simulink model "Level1"  (R2021a)
settings: Solver=VariableStepAuto  StartTime=0.0  StopTime=10.0  RelTol=1e-3
values from neighbouring files (symbols this model uses):
  ax_max = 0.8    [Data.m]
  ay_max = 0.75    [Data.m]
  Bseg = 2    [Data.m]
  containerLayout = [3 2 2 4 3 4 2 1 4]    [Data.m]
  containerWidth = 2.5    [Data.m]
  dx = 0.1    [Data.m]    (also in generate_profile.m)
  Hseg = 3    [Data.m]
  jerkh = 4    [Data.m]
  jerkt = 2    [Data.m]
  vx_max = 4    [Data.m]
  vy_loaded_max = 1.5    [Data.m]
  vy_unloaded_max = 3    [Data.m]
  x_axis = [-30 50]    [Data.m]
  X_bay = [-22,-15,-8]    [Data.m]
  X_container = [2.8,5.4,8,10.6,13.2,15.8,18.4,21,23.6]    [Data.m]
  y_axis = [-20 40]    [Data.m]
  Yt0 = 45    [Data.m]
libraries: simulink x1
settings Model: Creator=jpss8  LastModifiedBy=ThnkPad

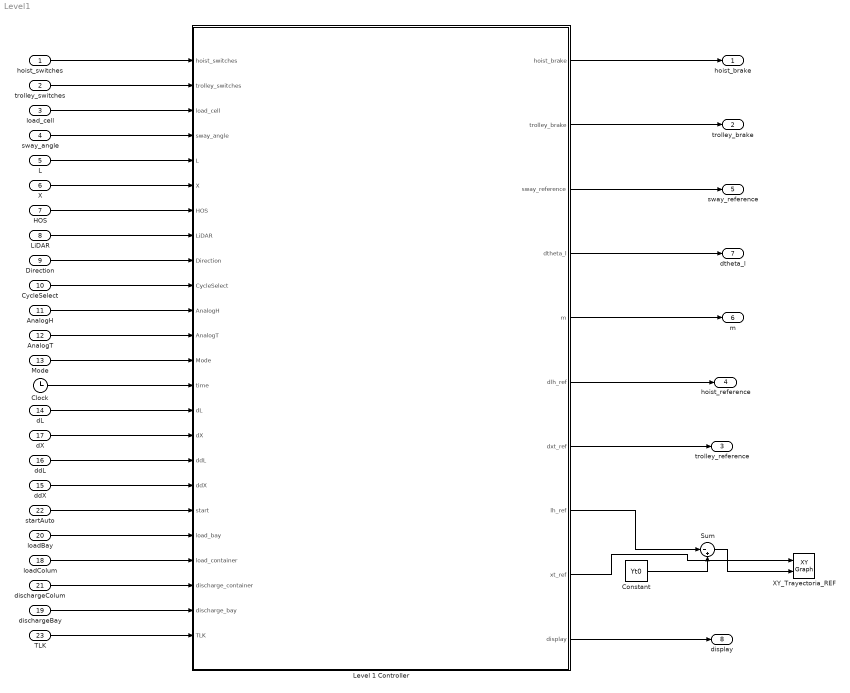
== system Level1 ==
  hoist_switches : Inport  PortDimensions=4
  trolley_switches : Inport  Port=2  PortDimensions=4
  load_cell : Inport  Port=3
  sway_angle : Inport  Port=4
  L : Inport  Port=5
  X : Inport  Port=6
  HOS : Inport  Port=7
  LiDAR : Inport  Port=8
  Direction : Inport  Port=9
  CycleSelect : Inport  Port=10
  AnalogH : Inport  Port=11
  AnalogT : Inport  Port=12
  Mode : Inport  Port=13
  dL : Inport  Port=14
  ddX : Inport  Port=15
  ddL : Inport  Port=16
  dX : Inport  Port=17
  loadColum : Inport  Port=18
  dischargeBay : Inport  Port=19
  loadBay : Inport  Port=20
  dischargeColum : Inport  Port=21
  startAuto : Inport  Port=22
  TLK : Inport  Port=23
  Clock : Clock
  Constant : Constant  Value=Yt0
  Level 1 Controller : Stateflow chart  TreatAsAtomicUnit=on
  Sum : Sum  Inputs=|-+
  XY_Trayectoria_REF : simulink/Sinks/XY Graph  xmin=-30  xmax=50  ymin=-20  ymax=45  st=-1
  hoist_brake : Outport
  trolley_brake : Outport  Port=2
  trolley_reference : Outport  Port=3
  hoist_reference : Outport  Port=4
  sway_reference : Outport  Port=5
  m : Outport  Port=6
  dtheta_l : Outport  Port=7
  display : Outport  Port=8
  wires:
  load_cell/1 -> Level 1 Controller/3(load_cell)
  sway_angle/1 -> Level 1 Controller/4(sway_angle)
  L/1 -> Level 1 Controller/5(L)
  Level 1 Controller/6(dlh_ref) -> hoist_reference/1
  Level 1 Controller/2(trolley_brake) -> trolley_brake/1
  Level 1 Controller/1(hoist_brake) -> hoist_brake/1
  Level 1 Controller/3(sway_reference) -> sway_reference/1
  HOS/1 -> Level 1 Controller/7(HOS)
  trolley_switches/1 -> Level 1 Controller/2(trolley_switches)
  hoist_switches/1 -> Level 1 Controller/1(hoist_switches)
  LiDAR/1 -> Level 1 Controller/8(LiDAR)
  Direction/1 -> Level 1 Controller/9(Direction)
  CycleSelect/1 -> Level 1 Controller/10(CycleSelect)
  AnalogH/1 -> Level 1 Controller/11(AnalogH)
  AnalogT/1 -> Level 1 Controller/12(AnalogT)
  Mode/1 -> Level 1 Controller/13(Mode)
  Level 1 Controller/5(m) -> m/1
  Level 1 Controller/4(dtheta_l) -> dtheta_l/1
  X/1 -> Level 1 Controller/6(X)
  Clock/1 -> Level 1 Controller/14(time)
  dL/1 -> Level 1 Controller/15(dL)
  Level 1 Controller/9(xt_ref) -> XY_Trayectoria_REF/1
  Sum/1 -> XY_Trayectoria_REF/2
  Level 1 Controller/8(lh_ref) -> Sum/1
  Constant/1 -> Sum/2
  Level 1 Controller/7(dxt_ref) -> trolley_reference/1
  dX/1 -> Level 1 Controller/16(dX)
  ddL/1 -> Level 1 Controller/17(ddL)
  ddX/1 -> Level 1 Controller/18(ddX)
  loadBay/1 -> Level 1 Controller/20(load_bay)
  loadColum/1 -> Level 1 Controller/21(load_container)
  dischargeColum/1 -> Level 1 Controller/22(discharge_container)
  dischargeBay/1 -> Level 1 Controller/23(discharge_bay)
  startAuto/1 -> Level 1 Controller/19(start)
  Level 1 Controller/10(display) -> display/1
  TLK/1 -> Level 1 Controller/24(TLK)

== stateflow chart Level1/Level 1 Controller ==
  state AutoSecuence [parallel]
    settings: executionOrder=3
    state stay
      entry:
      display=4;
      AUTO=0;
    state automaticSecuence
      state Positioning [group]
        state m1
          %manual hasta salir de manualZone
          entry:
          AUTO=0;
          display=0;
        state Pos
          entry:
          %ir hasta la bahia de carga seleccionada
          Xf=X_bay(discharge_bay);
          Yf=interp1(manualZone(1,:),manualZone(2,:), Xf, 'linear');
          AutoFlag=0;
          AUTO=1;
          display=1;
        state m2a
          entry:
          %tomar el container
          AUTO=0;
          display=2;
        m1 -> Pos : [MZF==0]
        Pos -> m2a : [AutoFlag==1]
      state go [group]
        state m2b
          %salir de la zona manual
          display=0;
        state Go
          entry:
          %ir hasta la culumna a cargar
          Xf=X_container(load_container);
          Yf=interp1(manualZone(1,:),manualZone(2,:), Xf, 'linear');
          AutoFlag=0;
          AUTO=1;
          display=1;
        state m3a
          entry:
          %soltar manualmente el container
          AUTO=0;
          display=3;
        m2b -> Go : [MZF==0]
        Go -> m3a : [AutoFlag==1]
      state Transit [group]
        state m3b
          %salir de la zona manual
          display=0;
        state Transist
          %ir hasta la columna de container a descargar
          entry:
          Xf=X_container(discharge_container);
          Yf=interp1(manualZone(1,:),manualZone(2,:), Xf, 'linear');
          AutoFlag=0;
          AUTO=1;
          display=1;
        state m4a
          %tomar el container manualmente
          entry:
          AUTO=0;
          display=2;
        AutoSecuence.automaticSecuence.Transit.m3b -> Transist : [MZF==0]
        Transist -> AutoSecuence.automaticSecuence.Transit.m4a : [AutoFlag==1]
      state Return [group]
        state m3b
          %salir de la zona manual para volver
          display=0;
        state Return
          %if hasta la bahia de carga a cargar
          entry:
          Xf=X_bay(load_bay);
          Yf=interp1(manualZone(1,:),manualZone(2,:), Xf, 'linear');
          AutoFlag=0;
          AUTO=1;
          display=1;
        state m4a
          entry:
          AUTO=0;
          display=3;
        AutoSecuence.automaticSecuence.Return.m3b -> AutoSecuence.automaticSecuence.Return.Return : [MZF==0]
        AutoSecuence.automaticSecuence.Return.Return -> AutoSecuence.automaticSecuence.Return.m4a : [AutoFlag==1]
      (default) -> m1
      m2a -> m2b : [TLK==1]
      m3a -> AutoSecuence.automaticSecuence.Transit.m3b : [TLK==0]
      AutoSecuence.automaticSecuence.Transit.m4a -> AutoSecuence.automaticSecuence.Return.m3b : [TLK==1]
    (default) -> stay
    automaticSecuence -> stay : [Mode==0]
    stay -> automaticSecuence : [Mode==1 && start==1]
  state ObstacleProfile [parallel]
    entry:
    obst_profile=ones(2,(x_axis(2)-x_axis(1))/dx+1);
    obst_profile(1,:)=[x_axis(1):dx:x_axis(2)];
    manualZone=obst_profile;
    obst_profile(2,:)=obst_profile(2,:)*15;%y_axis(2)-5;
    obst_profile=obsProfGen(containerLayout);%prueba!!!!!!!!!!!!!!!!!!!!!!!!!!!!!!!!!!!!!!!!!!!!!!!!!!!!!!
    MZF=1;
    k=1;
    during:
    if TLK==0
    while obst_profile(1,k+1)<X
    k=k+1;
    end
    while obst_profile(1,k-1)>X
    k=k-1;
    end
    obst_profile(2,k)=Yt0-LiDAR;
    end
    manualZone=ObsToManaualZone(Hseg,Bseg,obst_profile);
    if MZF==1
    if interp1(manualZone(1,:),manualZone(2,:), X, 'linear')+0.2<Yt0-L
    MZF=0;
    end
    else
    if interp1(manualZone(1,:),manualZone(2,:), X, 'linear')-0.2>Yt0-L
    MZF=1;
    end
    end
    settings: executionOrder=2
  state Main [parallel]
    settings: executionOrder=1
    state On
      entry:
      sway_reference = 0;
      m = 0;
      dtheta_l = 0;
      dxt_ref=0;
      dlh_ref=0;
    state Manual
      entry:
      AnalogH_1=0;
      jH=1;
      AnalogT_1=0;
      jT=1;
      t0H=time;
      t0T=time;
      if TLK==0
      vH_max=vy_unloaded_max;
      else
      vH_max=vy_loaded_max;
      end
      [t_H,v_H]= vel_prof_gen(-dL, -AnalogH*vH_max/100 , -ddL ,vH_max,ay_max, jerkh,0.0005);
      [t_T,v_T]= vel_prof_gen(dX, AnalogT*vx_max/100 , ddX ,vx_max,ax_max, jerkt,0.0005);
      during:
      %-----------------------HOIST---------------------------------------------------
      if abs(AnalogH-AnalogH_1)>abs(AnalogH)*0.01
      AnalogH_1=AnalogH;
      jH=1;
      t0H=time;
      if TLK==0
      vH_max=vy_unloaded_max;
      else
      vH_max=vy_loaded_max;
      end
      [t_H,v_H]= vel_prof_gen(-dL, -AnalogH*vH_max/100 , -ddL ,vH_max,ay_max, jerkh,0.0005);
      end
      if time>t0H+t_H(end)
      dlh_ref=-v_H(end);
      else
      while time>t_H(jH)+t0H
      jH=jH+1;
      end
      dlh_ref=-v_H(jH);
      end
      %------------------------TROLLEY---------------------------------------------
      if abs(AnalogT-AnalogT_1)>abs(AnalogT)*0.01
      AnalogT_1=AnalogT;
      jT=1;
      t0T=time;
      [t_T,v_T]= vel_prof_gen(dX, AnalogT*vx_max/100 , ddX ,vx_max,ax_max, jerkt,0.0005);
      end
      if time>t0T+t_T(end)
      dxt_ref=v_T(end);
      else
      while time>t_T(jT)+t0T
      jT=jT+1;
      end
      dxt_ref=v_T(jT);
      end
    state Automatic
      entry:
      Xf=X_bay(load_bay);
      Yf=interp1(manualZone(1,:),manualZone(2,:), Xf, 'linear');
      disp([X,Yt0-L])
      disp([Xf,Yf])
      disp(-dL)
      disp(vy_unloaded_max)
      disp(vx_max)
      disp(-ddL)
      if (TLK==0)
      [T_,Qhoist_,Qtrolley_]=traj_gen(obst_profile',[X,Yt0-L],[Xf,Yf],-dL,0,vy_unloaded_max,vx_max,0,0,ay_max,ax_max,jerkt,jerkh,containerWidth,Hseg);
      else
      [T_,Qhoist_,Qtrolley_]=traj_gen(obst_profile',[X,Yt0-L],[Xf,Yf],-dL,0,vy_loaded_max,vx_max,0,0,ay_max,ax_max,jerkt,jerkh,containerWidth,Hseg);
      end
      set(TrajP,'XData', Qtrolley_(1,:), 'YData', Qhoist_(1,:));
      t0=time;
      N=length(T_);
      i_=1;
      during:
      if time-t0>T_(end)
      AutoFlag=1;
      else
      while T_(i_)<time-t0
      i_=i_+1;
      end
      dlh_ref=-Qhoist_(2,i_);
      dxt_ref=Qtrolley_(2,i_);
      lh_ref=Yt0-Qhoist_(1,i_);
      xt_ref=Qtrolley_(1,i_);
      end
    (default) -> On
    On -> Manual
    Automatic -> Manual : [AUTO==0]
    Manual -> Automatic : [AUTO==1]
  state Breaks [parallel]
    during:
    if dxt_ref==0
    trolley_brake = 0;
    else
    trolley_brake = 0;
    end
    if dlh_ref==0
    hoist_brake = 0;
    else
    hoist_brake = 0;
    end
    settings: executionOrder=5
  note: ?
  state Plot [parallel]
    entry:
    close all;
    figure(1);
    h = plot(nan, nan);
    hold on;
    TrajP = plot(nan, nan,'r');
    p = plot(nan, nan, 'ro', 'MarkerFaceColor', 'r');
    ps = plot(nan, nan, 'ro', 'MarkerFaceColor', 'b');
    xlabel('Eje X');
    ylabel('Eje Y');
    title('Grafico XY Animado');
    xlim([-30, 50]);
    ylim([-20, 45]);
    during:
    set(h, 'XData', obst_profile(1,:), 'YData', obst_profile(2,:));
    set(p, 'XData', X, 'YData', Yt0);
    set(ps, 'XData', X, 'YData', Yt0-L);
    drawnow;
    settings: executionOrder=4
  data: ManualZone function_output; hseg function_input; bseg function_input; obsProfile function_input; O_profile function_input; P0 function_input; Pf function_input; v0h function_input; vfh function_input; vmaxh function_input; vmaxt function_input; a0h function_input; afh function_input; amaxh function_input; amaxt function_input; T function_output; Qhoist function_output; Qtrolley function_output; jt function_input; jh function_input; xbox function_input; hseg function_input; Ob_profile function_output; Layout function_input; v0 function_input; vc function_input; a0 function_input; v_max function_input; a_max function_input; J function_input; dt function_input; t function_output; v function_output; hoist_brake output; trolley_brake output; hoist_switches input; trolley_switches input; load_cell input; sway_angle input; L input; X input; sway_reference output; dtheta_l output; HOS input; LiDAR input; Direction input; CycleSelect input; AnalogH input; AnalogT input; Mode input; m output; time input; t0 local; vy_loaded_max parameter; vy_unloaded_max parameter; ax_max parameter; vx_max parameter; ay_max parameter; dL input; i local; obst_profile local size=[2 801]; Qtrolley_ local size=[4 10000000]; T_ local size=[1 10000000]; Qhoist_ local size=[4 10000000]; jerkh parameter; jerkt parameter; containerWidth parameter; Hseg parameter; Yt0 parameter; dlh_ref output; dxt_ref output; lh_ref output; xt_ref output; N local; dX input; al_1 local; ax_1 local; t_1 local; Dt local; ddL input; ddX input; a_H local; a_T local; jT local; jH local; t0H local; vH_max local; t_H local size=10000000; v_H local size=10000000; t0T local; t_T local size=10000000; v_T local size=10000000; AnalogH_1 local; AnalogT_1 local; start input; X_bay parameter; load_bay input; dx parameter; x_axis parameter; y_axis parameter; load_container input; discharge_container input; X_container parameter; discharge_bay input; display output int8; manualZone local size=[2 801]; Xf local; Yf local; AutoFlag local; MZF local; Bseg parameter; AUTO local; TLK input; k local; i_ local; h local; containerLayout parameter size=9; p local; TrajP local; ps local
  function ManualZone=ObsToManaualZone(hseg,bseg,obsProfile):
    | function ManualZone=ObsToManaualZone(hseg,bseg,obsProfile)
    | 
    | ManualZone=obsProfile;
    | ManualZone(2,:)=obsProfile(2,:)+hseg;
    | 
    | N=round(bseg/(obsProfile(1,2)-obsProfile(1,1)));
    | 
    | for i=1:N
    |     ManualZone(2,i)=max(obsProfile(2,1:i+N)); 
    | end
    | for i=1+N:length(obsProfile(2,:))-N
    |     ManualZone(2,i)=max(obsProfile(2,i-N:i+N)); 
    | end
    | for i=length(obsProfile(2,:))-N+1:length(obsProfile(2,:))
    |     ManualZone(2,i)=max(obsProfile(2,i-N:end)); 
    | end
    | 
    | ManualZone(2,:)=ManualZone(2,:)+hseg;
    | 
    | end
  function [T,Qhoist,Qtrolley]=traj_gen(O_profile,P0,Pf,v0h,vfh,vmaxh,vmaxt,a0h,afh,amaxh,amaxt,jt,jh,xbox,hseg):
    | 
    | 
    | function [T,Qhoist,Qtrolley]=traj_gen(O_profile,P0,Pf,v0h,vfh,vmaxh,vmaxt,a0h,afh,amaxh,amaxt,jt,jh,xbox,hseg)
    | % Esta función genera una trayectoria para un sistema de elevación, como un
    | % montacargas o una grúa, en función de un perfil de elevación dado. 
    | % La trayectoria contempla aceleración con perfil trapeziodal.
    | % Busca generar una trayectoria eficiente donde evite los obstaculos con un
    | % marquen dado.
    | % Además admite casos donde la la aceleracion maxima o la velocidad maxima sean
    | % mayores a las posible para un determinado recorrido. Estos casos de
    | % diminuye automaticamente su valor para cumplir con los otros
    | % requirimientos.
    | %
    | % Argumentos de entrada:
    | % - O_profile: matriz que contiene el perfil de elevación. Cada fila representa
    | %   un punto en el perfil, donde la primera columna contiene las coordenadas
    | %   horizontales y la segunda columna contiene las alturas correspondientes.
    | % - P0: punto inicial de la trayectoria, dado como [x0, y0].
    | % - Pf: punto final de la trayectoria, dado como [xf, yf].
    | % - v0h: velocidad inicial de elevación.
    | % - vfh: velocidad final de elevación.
    | % - vmaxh: velocidad máxima de elevación.
    | % - vmaxt: velocidad máxima de desplazamiento horizontal.
    | % - a0h: aceleración inicial de elevación.
    | % - afh: aceleración final de elevación.
    | % - amaxh: aceleración máxima de elevación.
    | % - amaxt: aceleración máxima de desplazamiento horizontal.
    | %
    | % Las siguientes variables se toman del espacio de trabajo (workspace):
    | % - hseg: altura de seguridad adicional a considerar.
    | % - xbox: distancia horizontal alrededor de los puntos iniciales y finales
    | %   para buscar el perfil.
    | % - jh: jerk máximo permitido en la elevación.
    | % - jt: jerk máximo permitido en el desplazamiento horizontal.
    | %
    | % Argumentos de salida:
    | % - T: vector de tiempo de la trayectoria generada.
    | % - Qhoist: matriz que describe la trayectoria de elevación generada.
    | %   Siento las filas Q(1,:) la posición, Q(2,:) la velocidad,
    | %   Q(3,:)aceleracion y Q(4,:) el jerk
    | % - Qtrolley: matriz que describe la trayectoria de desplazamiento horizontal
    | %   generada. misma estructura que Qtrolley
    |     
    |     
    |     %Caso degenerado=======================================================
    |     if P0(1)==Pf(1)
    |         [T,Qhoist] = trap_acc_prof(P0(2),Pf(2),v0h,0,a0h,0,vmaxh,amaxh,jh);
    |         Qtrolley=zeros(4,length(T));
    |         Qtrolley(1,:)=ones(1,length(T))*P0(1);
    |         return;
    |     end  
    | 
    |     %=========================================================================
    |     %Calculo de puntos
    |     %=========================================================================
    |     %recortar O_profile entre x0 y xf (O_profile_r)
    |     O_profile_r=subO_profile(O_profile,P0(1),Pf(1));
    | 
    |     %Hmax es igual a la altula maxima en O_profile_r mas una altura de seguridad "h_seg"
    |     Hmax=max(O_profile_r(:,2))+hseg;
    | 
    |     %H0 es la altura que parte de Y0 y termina cuando el O_profile es superado en
    |     %un entorno de 1.5 xbox de X0 mas h_seg.
    |     H0=max(subO_profile(O_profile,P0(1)-xbox*1.5,P0(1)+xbox*1.5))+hseg;
    |     H0=H0(2);
    |     %H1 lo mismo
    |     Hf=max(subO_profile(O_profile,Pf(1)-xbox*1.5,Pf(1)+xbox*1.5))+hseg;
    |     Hf=Hf(2);
    |     %se traza una recta entre xo y el se la hace "tangente" (que solo toca un 
    |     %punto del O_profile)
    | 
    |     if Pf(1)>P0(1)
    |         xl=P0(1);
    |         xh=Pf(1);
    |         Hl=H0;
    |         Hh=Hf;
    |     else
    |         xh=P0(1);
    |         xl=Pf(1);
    |         Hh=H0;
    |         Hl=Hf;
    |     end
    | 
    |     mmax=0;
    |     prof=subO_profile(O_profile,xl+xbox*0.5,inf);
    |     for i=1:length(prof)
    |         if prof(i,2)+hseg<Hl
    |             continue
    |         end
    |         if (prof(i,2)+hseg-Hl)/(prof(i,1)-xbox-xl(1))>mmax
    |             mmax=(prof(i,2)-Hl+hseg)/(prof(i,1)-xl(1)-xbox);
    |         end
    |     end
    |     DXl=(Hmax-Hl)/mmax;
    | 
    |     mmax=0;
    |     prof=subO_profile(O_profile,xh-xbox*0.5,-inf);
    |     for i=1:length(prof)
    |         if prof(i,2)+hseg<Hh
    |             continue
    |         end
    |         if (prof(i,2)+hseg-Hh)/(prof(i,1)+xbox-xh(1))<mmax
    |             mmax=(prof(i,2)-Hh+hseg)/(prof(i,1)-xh(1)+xbox);
    |         end
    |     end
    |     DXh=(Hmax-Hh)/mmax;
    | 
    |     if Pf(1)>P0(1)
    |         x02=P0(1)+DXl;
    |         xf2=Pf(1)+DXh;
    |     else
    |         x02=P0(1)+DXh;
    |         xf2=Pf(1)+DXl;
    |     end
    | 
    |     %graficar
    |     %figure(10)
    |     %plot(O_profile(:,1),O_profile(:,2))
    |     %hold on
    |     %plot(O_profile_r(:,1),O_profile_r(:,2))
    |     %plot(x02,Hmax,'x')
    |     %plot(xf2,Hmax,'x')
    |     %plot(P0(1),H0,'x')
    |     %plot(Pf(1),Hf,'x')
    |     %plot(P0(1),P0(2),'x')
    |     %plot(Pf(1),Pf(2),'x')
    | 
    |     %end
    |     %=========================================================================
    |     %Calculo de trayectoria
    |     %=========================================================================
    |     %trap_acc_prof(p0, pf, v0, vf, a0, af, vmax, amax, jk)
    |     %disp("raise---------------------------")
    |     [Traise,Qraise] = trap_acc_prof(P0(2),Hmax,v0h,0,a0h,0,vmaxh,amaxh,jh);
    |     %disp("lower-------------------------------")
    |     [Tlower,Qlower] = trap_acc_prof(Hmax,Pf(2),0,vfh,0,afh,vmaxh,amaxh,jh);
    |     %disp("slide----------------------")
    |     [Tslide, Qslide] = trap_acc_prof(P0(1),Pf(1),0,0,0,0,vmaxt,amaxt,jt);
    |     %disp("----")
    | 
    |     % Configuración de los subplots
    | %     num_plots = size(Qslide, 1); % Número de vectores en Qslide
    | %     num_rows = ceil(sqrt(num_plots)); % Número de filas de subplots
    | %     num_cols = ceil(num_plots / num_rows); % Número de columnas de subplots
    | 
    |     % Crear figura para subplots
    | %     figure;
    | % 
    | %     % Plotear los vectores Qslide utilizando subplots
    | %     for i = 1:num_plots
    | %         subplot(num_rows, num_cols, i);
    | %         plot(Tslide, Qslide(i, :));
    | %         title(['Qslide(', num2str(i), ', :)']);
    |     %    xlabel('Tiempo');
    |     %    ylabel('Qslide');
    |     %end
    |     %disp(Qlower(1,:))
    |     %figure(2)
    |     %plot(Tlower,Qlower(1,:))
    |     %figure(3)
    |     %plot(Tlower,Qlower(2,:))
    |     %figure(4)
    |     %plot(Tlower,Qlower(3,:))
    |     %figure(5)
    |     %plot(Tlower,Qlower(4,:))
    |     %-----------------------------------------------------------------------
    |     N0x=time_between(Qslide(1,:),Tslide,P0(1),x02);
    |     N0y=time_between(Qraise(1,:),Traise,Hmax,H0);
    | 
    |     if N0y>N0x
    |         Qtrolley=zeros(4,length(Traise)-N0x);
    |         Qtrolley(1,:)=Qslide(1,1);
    |         Qtrolley=[Qtrolley Qslide];
    |         T=[Traise(1:length(Traise)-N0x) Tslide+Traise(length(Traise)-N0x)];
    |     else
    |         Qtrolley=zeros(4,length(Traise)-N0y);
    |         Qtrolley(1,:)=Qslide(1,1);
    |         Qtrolley=[Qtrolley Qslide];
    |         T=[Traise(1:length(Traise)-N0y) Tslide+Traise(length(Traise)-N0y)];
    |     end
    |     %-----------------------------------------------------------------------
    |     Nfx=time_between(Qslide(1,:),Tslide,Pf(1),xf2);
    |     Nfy=time_between(Qlower(1,:),Tlower,Hmax,Hf);
    | 
    |     if Nfx>Nfy
    |         aux=zeros(4,length(Tlower)-Nfy);
    |         aux(1,:)=Qslide(1,end);
    |         Qtrolley=[Qtrolley aux];
    |         T=[T T(end)+Tlower(1:length(Tlower)-Nfy)];
    |     else
    |         aux=zeros(4,length(Tlower)-Nfx);
    |         aux(1,:)=Qslide(1,end);
    |         Qtrolley=[Qtrolley aux];
    |         T=[T T(end)+Tlower(1:length(Tlower)-Nfx)];
    |     end
    |     
    |     %-----------------------------------------------------------------------
    |     Qhoist=zeros(4,length(Qtrolley)-length(Qlower)-length(Qraise));
    |     Qhoist(1,:)=Hmax;
    |     Qhoist=[Qraise Qhoist Qlower];
    | end
    | 
    | 
    | 
    | 
    | 
    | 
    | function [T,Q] = trap_acc_prof(p0, pf, v0, vf, a0, af, vmax, amax, jk)
    |     if p0>pf
    |         vmax=-vmax;
    |         amax=-amax;
    |         jk=-jk;    
    |     end
    |     amax0=amax;
    |     amaxf=amax;
    |   
    |     [t1,t2,t3,t4,t5,t6,t7]=times_trap_acc_prof(p0, pf, v0, vf, a0, af, vmax, amax0, amaxf, jk);
    |     
    | 
    |         while t2<0
    |             amax0=amax0*0.99;
    |             [t1,t2,t3,t4,t5,t6,t7]=times_trap_acc_prof(p0, pf, v0, vf, a0, af, vmax, amax0, amaxf, jk);
    |         end
    |         if t2<=0
    |             a=-1/jk;
    |             c=vmax-v0+a0^2/jk/2;
    |             amax0=sign(amax)*abs(sqrt(- 4 * a * c) / 2 / a);
    |             [t1,t2,t3,t4,t5,t6,t7]=times_trap_acc_prof(p0, pf, v0, vf, a0, af, vmax, amax0, amaxf, jk);   
    |         end
    | 
    |         if t6<=0
    |             a=1/jk;
    |             c=vf-vmax-af^2/jk/2;
    |             amaxf=sign(amax)*abs(sqrt(- 4 * a * c) / 2 / a);
    |             [t1,t2,t3,t4,t5,t6,t7]=times_trap_acc_prof(p0, pf, v0, vf, a0, af, vmax, amax0, amaxf, jk);   
    |         end
    |         
    |         while t2<0 || t6<0 ||t4<0
    |             if t2<0
    |                 amax0=amax0*0.97;
    |             end
    |             if t6<0
    |                 amaxf=amaxf*0.97;
    |             end
    |             if t4<0
    |                 vmax=vmax*0.97;
    |             end
    |                 
    |             [t1,t2,t3,t4,t5,t6,t7]=times_trap_acc_prof(p0, pf, v0, vf, a0, af, vmax, amax0, amaxf, jk);   
    |         end
    | 
    | 
    | 
    | dt=0.00001;
    | T1=0:sign(t1)*dt:t1;
    | T2=0:sign(t2)*dt:t2;
    | T3=0:sign(t3)*dt:t3;
    | T4=0:sign(t4)*dt:t4;
    | T5=0:sign(t5)*dt:t5;
    | T6=0:sign(t6)*dt:t6;
    | T7=0:sign(t7)*dt:t7;
    | 
    | 
    | Q1=zeros(4,length(T1));
    | Q2=zeros(4,length(T2));
    | Q3=zeros(4,length(T3));
    | Q4=zeros(4,length(T4));
    | Q5=zeros(4,length(T5));
    | Q6=zeros(4,length(T6));
    | Q7=zeros(4,length(T7));
    | 
    | 
    | for i=1:length(T1)
    | Q1(:,i)=const_j(p0,v0,a0,jk,T1(i));
    | end
    | for i=1:length(T2)
    | Q2(:,i)=const_j(Q1(1,end),Q1(2,end),amax0,0,T2(i));
    | end
    | 
    | for i=1:length(T3)
    | Q3(:,i)=const_j(Q2(1,end),Q2(2,end),amax0,-jk,T3(i));
    | end
    | for i=1:length(T4)
    | Q4(:,i)=const_j(Q3(1,end),vmax,0,0,T4(i));
    | end
    | for i=1:length(T5)
    | Q5(:,i)=const_j(Q4(1,end),vmax,0,-jk,T5(i));
    | end
    | for i=1:length(T6)
    | Q6(:,i)=const_j(Q5(1,end),Q5(2,end),-amaxf,0,T6(i));
    | end
    | for i=1:length(T7)
    | Q7(:,i)=const_j(Q6(1,end),Q6(2,end),-amaxf,jk,T7(i));
    | end
    |  
    |  Q=[Q1 Q2 Q3 Q4 Q5 Q6 Q7];
    |  
    |  T=[T1 T2+t1 T3+t1+t2 T4+t1+t2+t3 T5+t1+t2+t3+t4 T6+t1+t2+t3+t4+t5 T7+t1+t2+t3+t4+t5+t6];
    | 
    | end
    | 
    | 
    | function [t1,t2,t3,t4,t5,t6,t7] = times_trap_acc_prof(p0, pf, v0, vf, a0, af, vmax, amax0, amaxf, jk)
    | 
    |  %Etapa 1 - jerk constante 
    |     t1=(amax0-a0)/jk;
    |     v1=v0+a0*t1+0.5*jk*t1^2;
    |     p1=p0+v0*t1+0.5*a0*t1^2+(1/6)*jk*t1^3;
    | 
    |  %Etapa 3 - jkerk constante
    |     t3=amax0/jk;
    |     v2=vmax-amax0*t3+0.5*jk*t3^2;
    |     %p3=?
    |     
    |  %Etapa 2 - aceleracion constante
    |     t2=(v2-v1)/amax0;
    |     p2=p1+v1*t2+0.5*amax0*t2^2;
    |     %etapa 3
    |     p3=p2+v2*t3+0.5*amax0*t3^2-(1/6)*jk*t3^3;
    |  
    |  %Etapa 7 - jerk constante
    |     t7=(af-(-amaxf))/jk;
    |     v6=vf+amaxf*t7-0.5*jk*t7^2;
    |     p6=pf-v6*t7+0.5*amaxf*t7^2-(1/6)*jk*t7^3; 
    |  
    |  %Etapa 5 - jerk constante
    |     t5=amaxf/jk;
    |     v5=vmax-0.5*jk*t5^2;
    |     %p4=?
    |     
    |  %Etapa 6 - aceleracion constante
    |     t6=(v6-v5)/-amaxf;
    |     p5=p6-v5*t6+0.5*amaxf*t6^2;
    |     %etapa 5
    |     p4=p5-vmax*t5+(1/6)*jk*t5^3;
    | 
    |  %Etapa 4 - velocidad constante
    |     t4=(p4-p3)/vmax;
    |  
    | end
    | 
    | 
    | function Q=const_j(p0,v0,a0,jk,t)
    | Q=zeros(4,1);
    | Q(4)=jk;
    | Q(3)=a0+jk*t;
    | Q(2)=v0+a0*t+0.5*jk*t^2;
    | Q(1)=p0+v0*t+0.5*a0*t^2+(1/6)*jk*t^3;
    | 
    |  
    | end
    | 
    | function num_puntos = time_between(Q, ~, x0, x1)
    |     % Encontrar el índice más cercano a x0 en Q
    |     [~, i0] = min(abs(Q - x0));
    |     
    |     % Verificar si x0 es menor o mayor que el valor correspondiente en Q
    |     if x0 < Q(i0)
    |         i0 = i0 - 1;
    |     end
    |     
    |     % Encontrar el índice más cercano a x1 en Q
    |     [~, i1] = min(abs(Q - x1));
    |     
    |     % Verificar si x1 es menor o mayor que el valor correspondiente en Q
    |     if x1 < Q(i1)
    |         i1 = i1 - 1;
    |     end
    |     
    |     % Calcular la cantidad de puntos entre las posiciones x0 y x1
    |     num_puntos = abs(i1 - i0);
    | end
    | 
    | 
    | 
    | 
    | 
    | 
    | 
    | 
    | 
    | 
    | function subprof=subO_profile(vector,x0,xf)
    |     if x0>xf
    |         xmin=xf;
    |         xmax=x0;
    |     else
    |         xmin=x0;
    |         xmax=xf;
    |     end
    |     imin=1;
    |     while vector(imin,1)<xmin
    |         imin=imin+1;
    |         if imin>=length(vector(:,1))
    |             break
    |         end
    |     end
    |     imax=length( vector(:,1));
    |     while vector(imax,1)>xmax
    |         imax=imax-1;
    |         if imin<=1
    |             break
    |         end
    |     end
    |     subprof=vector(imin:imax,:);
    | end
  function Ob_profile=obsProfGen(Layout):
    | function Ob_profile=obsProfGen(Layout)
    | %% CONTAINER PROFILE -- constant container height = 2.5m
    |     cols = length(Layout);
    |     
    | 
    |     containerWidth_ = 2.5;
    |     xmin = -30;
    |     xmax = 50;
    |     N = (xmax - xmin)/0.1 + 1;
    |     Ob_profile = zeros(N,2);
    |     Ob_profile(:,1) = (xmin:0.1:xmax)';
    |     
    |     % Loading Bay1 - Bahia de carga 
    |     Ob_profile=ObstUpdate(Ob_profile,-23.5,-20.5,1);
    |     
    |     % Loading Bay2 - Bahia de carga 
    |     Ob_profile=ObstUpdate(Ob_profile,-16.5,-13.5,1);
    |     
    |     % Loading Bay3 - Bahia de carga 
    |     Ob_profile=ObstUpdate(Ob_profile,-9.5,-6.5,1);
    |     
    |     % Sill Beam - Viga Grua
    |     Ob_profile=ObstUpdate(Ob_profile,-2,0,15);
    |     
    |     % Gap 
    |     Ob_profile=ObstUpdate(Ob_profile,0,0.5,-2);
    |     
    |     % Ship wall - Pared barco
    |     Ob_profile=ObstUpdate(Ob_profile,0.5,1.5,5);
    |     
    |     % Ship floor - Piso barco
    |     Ob_profile=ObstUpdate(Ob_profile,1.5,24.9,-19);
    |     
    |     % Container stack
    |     for i=1:cols
    |         Ob_profile=ObstUpdate(Ob_profile,1.5+(i-1)*2.6,1.5+i*2.6,Layout(i)*2.4-19);
    |     end
    |     
    |     % Ship wall - Pared barco
    |     Ob_profile=ObstUpdate(Ob_profile,24.9,25.9,5);
    |     
    |     Ob_profile=Ob_profile';
    | end
    | 
    | function NewProfile=ObstUpdate(OldProfile,x0,x1,y)
    | NewProfile=OldProfile;
    | i=1;
    | while NewProfile(i,1)<x0
    |     i=i+1;
    | end
    | while NewProfile(i,1)<x1
    |     i=i+1;
    |     NewProfile(i,2)=y;
    | end
    | end
  function [t,v] = vel_prof_gen(v0, vc , a0 ,v_max,a_max, J,dt):
    | 
    | 
    | function [t,v] = vel_prof_gen(v0, vc , a0 ,v_max,a_max, J,dt)
    |     
    |     if abs(vc)>v_max
    |         vc=v_max*vc/abs(vc);
    |     end
    |     if v0>vc
    |         v_max=-v_max;
    |         a_max=-a_max;
    |         J=-J;    
    |     end
    | 
    |     [t1,t2,t3] = times_vel_prof_gen(v0, vc , a0 ,v_max,a_max, J);
    |     while t2<0
    |         a_max=a_max*0.99;
    |         [t1,t2,t3] = times_vel_prof_gen(v0, vc , a0 ,v_max,a_max, J);
    |     end
    | 
    |     T1=0:dt:t1;
    |     T2=0:dt:t2;
    |     T3=0:dt:t3;
    | 
    |     [V1, A1]=const_j(v0,a0,J,T1);
    |     if length(V1)~=0
    |         [V2, A2]=const_j(V1(end),a_max,0,T2);
    |     else
    |         [V2, A2]=const_j(v0,a_max,0,T2);
    |     end
    |     [V3, A3]=const_j(V2(end),a_max,-J,T3);
    |     
    |     v=[V1 V2 V3]';
    |     t=[T1 t1+T2 t1+t2+T3]';
    | 
    | end
    | 
    | function [v,a]=const_j(v0,a0,jk,t)
    | a=a0+jk.*t;
    | v=v0+a0.*t+0.5.*jk.*t.^2;
    | end
    | 
    | 
    | function [t1,t2,t3] = times_vel_prof_gen(v0, vc , a0 ,v_max,a_max, J)
    |   
    | t1=(a_max-a0)/J;
    | t3=a_max/J;
    | 
    | v1=v0+a0*t1+0.5*J*t1^2;
    | v2=vc-a_max*t3+0.5*J*t3^2;
    | 
    | t2=(v2-v1)/a_max;
    |     
    | end
